simulink model "pulse1"  (R2014b)
settings: Solver=ode45  StartTime=0.0  StopTime=0.5  MaxStep=.00001  RelTol=1e-3
libraries: simulink_extras x6, arduinolib x6, simulink x4, powerlib x1
settings Model: Creator=Muruganandham  LastModifiedBy=SELVA
settings DataIOCC: SignalLoggingSaveFormat=ModelDataLogs
settings OptimizationCC: ExpressionDepthLimit=2147483647
settings DebuggingCC: UnderspecifiedInitializationDetection=Classic  MergeDetectMultiDrivingBlocksExec=none  FcnCallInpInsideContextMsg=UseLocalSettings  StateNameClashWarn=warning
settings GRTTargetCC: CombineOutputUpdateFcns=off  GRTInterface=on

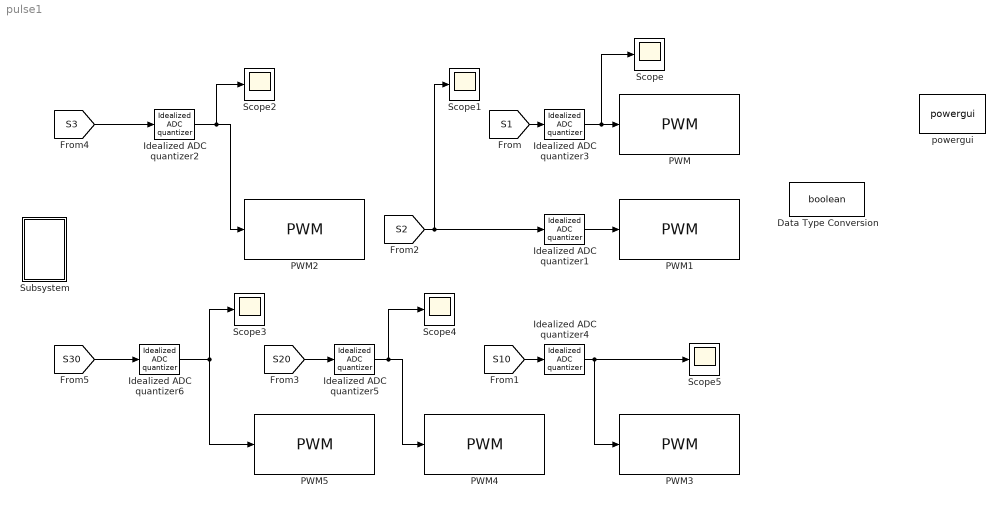
== system pulse1 ==
  Data Type Conversion : DataTypeConversion  OutDataTypeStr=boolean
  Idealized ADC quantizer{1..6} (6 alike) : simulink_extras/Additional Discrete/Idealized ADC quantizer  NumberOfConverterBits=8  Vmin=0  Vmax=5  OutputDataType=int16  OutputNegativeValues=off
  PWM : arduinolib/PWM  pinNumber=2  blockPlatform=arduino
  PWM1 : arduinolib/PWM  pinNumber=3  blockPlatform=arduino
  PWM2 : arduinolib/PWM  pinNumber=4  blockPlatform=arduino
  PWM3 : arduinolib/PWM  pinNumber=5  blockPlatform=arduino
  PWM4 : arduinolib/PWM  pinNumber=6  blockPlatform=arduino
  PWM5 : arduinolib/PWM  pinNumber=6  blockPlatform=arduino
  Scope{,1..5} (6 alike) : Scope
      Scope2 settings: SaveName=ScopeData2
      Scope3 settings: SaveName=ScopeData3
      Scope4 settings: SaveName=ScopeData4
      Scope5 settings: SaveName=ScopeData5
  Subsystem : Subsystem  mask{fc=1000, m=1}
      mask prompts: fc "Switching frequency"; m "modulation index"
  powergui : powerlib/powergui  Priority=1  SimulationMode=Continuous  SolverType=Tustin  SampleTime=50e-6  frequency=60  SPID=off  DisableSnubberDevices=off  DisableRonSwitches=off  DisableVfSwitches=off  SwTol=0  DisplayEquations=off  Interpol=off  methode=off  Ts=0  frequencyindice=0  Pbase=100e6  ErrMax=1e-4  Iterations=50  UnitsV=kV  UnitsW=MW  FunctionMessages=off  echomessages=off  HookPort=off  EnableUseOfTLC=off  x0status=blocks  RestoreLinks=warning  ResistiveCurrentMeasurement=off  Frange=[0:2:500]  Ylog=off  Xlog=on  ShowGrid=off  save=off  variable=ZData  structure=bh  ZoomFFT=off  StartTime=0.0  cycles=50  DisplayStyle=1  fundamental=50  FreqAxis=off  MaxFrequency=1000  frequencyindicesteady=1  RmsSteady=1  display=off
  wires:
  [S1] -> Idealized ADC quantizer3/1
  [S2] -> Scope1/1, Idealized ADC quantizer1/1
  [S3] -> Idealized ADC quantizer2/1
  [S10] -> Idealized ADC quantizer4/1
  [S20] -> Idealized ADC quantizer5/1
  [S30] -> Idealized ADC quantizer6/1
  Idealized ADC quantizer2/1 -> Scope2/1, PWM2/1
  Idealized ADC quantizer1/1 -> PWM1/1
  Idealized ADC quantizer3/1 -> Scope/1, PWM/1
  Idealized ADC quantizer4/1 -> Scope5/1, PWM3/1
  Idealized ADC quantizer5/1 -> Scope4/1, PWM4/1
  Idealized ADC quantizer6/1 -> Scope3/1, PWM5/1

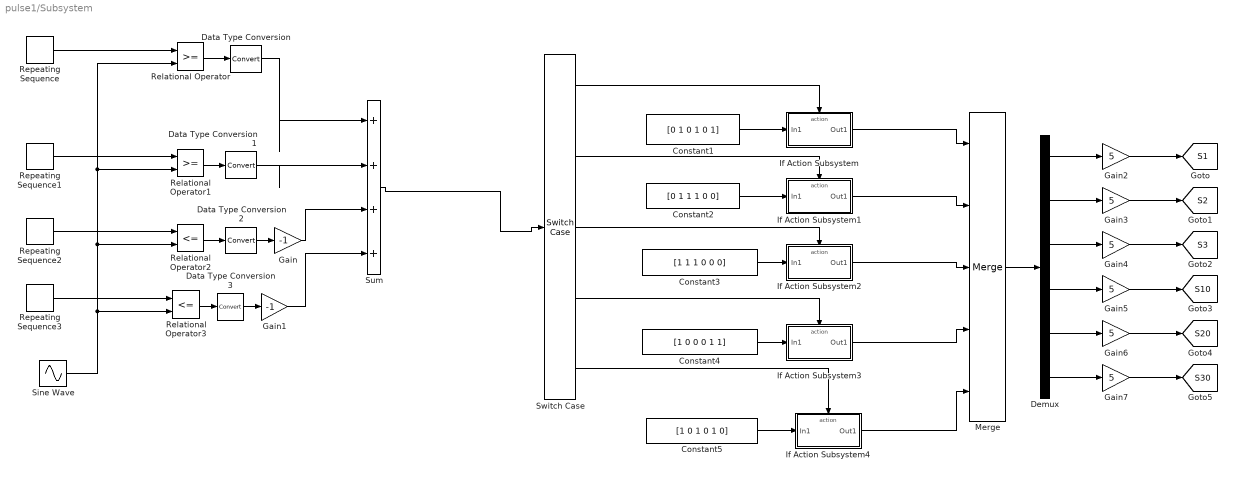
== system pulse1/Subsystem ==
  Constant1 : Constant  Value=[0 1 0 1 0 1]
  Constant2 : Constant  Value=[0 1 1 1 0 0]
  Constant3 : Constant  Value=[1 1 1 0 0 0]
  Constant4 : Constant  Value=[1 0 0 0 1 1]
  Constant5 : Constant  Value=[1 0 1 0 1 0]
  Data Type Conversion{,1..3} (4 alike) : DataTypeConversion
  Demux : Demux  Outputs=6
  Gain : Gain  Gain=-1
  Gain1 : Gain  Gain=-1
  Gain{2..7} (6 alike) : Gain  Gain=5
  If Action Subsystem : Subsystem  TreatAsAtomicUnit=on
  If Action Subsystem1 : Subsystem  TreatAsAtomicUnit=on
  If Action Subsystem2 : Subsystem  TreatAsAtomicUnit=on
  If Action Subsystem3 : Subsystem  TreatAsAtomicUnit=on
  If Action Subsystem4 : Subsystem  TreatAsAtomicUnit=on
  Merge : Merge  Inputs=5
  Relational Operator : RelationalOperator  OutDataTypeStr=boolean
  Relational Operator1 : RelationalOperator  OutDataTypeStr=boolean
  Relational Operator2 : RelationalOperator  Operator=<=  OutDataTypeStr=boolean
  Relational Operator3 : RelationalOperator  Operator=<=  OutDataTypeStr=boolean
  Repeating Sequence : simulink/Sources/Repeating Sequence  rep_seq_t="[0 (1/fc)/2  (1/fc)]"  rep_seq_y=[1 2 1]
  Repeating Sequence1 : simulink/Sources/Repeating Sequence  rep_seq_t="[0 (1/fc)/2  (1/fc)]"  rep_seq_y=[1 0 1]
  Repeating Sequence2 : simulink/Sources/Repeating Sequence  rep_seq_t="[0 (1/fc)/2  (1/fc)]"  rep_seq_y=[-1 0 -1]
  Repeating Sequence3 : simulink/Sources/Repeating Sequence  rep_seq_t="[0 (1/fc)/2  (1/fc)]"  rep_seq_y=[-1 -2 -1]
  Sine Wave : Sin  Amplitude=2*m  Frequency=2*pi*50  SampleTime=0
  Sum : Sum  Inputs=|++++
  Switch Case : SwitchCase  CaseConditions={-2 -1 0 1 2}  ShowDefaultCase=off
  tag scope: S10=global, S1=global, S20=global, S2=global, S30=global, S3=global
  wires:
  Switch Case/5 -> If Action Subsystem4/Action
  Switch Case/4 -> If Action Subsystem3/Action
  Switch Case/3 -> If Action Subsystem2/Action
  Switch Case/2 -> If Action Subsystem1/Action
  Switch Case/1 -> If Action Subsystem/Action
  Constant1/1 -> If Action Subsystem/1(In1)
  Constant2/1 -> If Action Subsystem1/1(In1)
  Constant3/1 -> If Action Subsystem2/1(In1)
  Constant4/1 -> If Action Subsystem3/1(In1)
  Constant5/1 -> If Action Subsystem4/1(In1)
  If Action Subsystem/1(Out1) -> Merge/1
  If Action Subsystem1/1(Out1) -> Merge/2
  If Action Subsystem2/1(Out1) -> Merge/3
  If Action Subsystem3/1(Out1) -> Merge/4
  If Action Subsystem4/1(Out1) -> Merge/5
  Merge/1 -> Demux/1
  Demux/2 -> Gain3/1
  Demux/3 -> Gain4/1
  Demux/4 -> Gain5/1
  Demux/5 -> Gain6/1
  Demux/6 -> Gain7/1
  Relational Operator/1 -> Data Type Conversion/1
  Relational Operator1/1 -> Data Type Conversion1/1
  Gain/1 -> Sum/3
  Gain1/1 -> Sum/4
  Sum/1 -> Switch Case/1
  Repeating Sequence/1 -> Relational Operator/1
  Repeating Sequence1/1 -> Relational Operator1/1
  Repeating Sequence2/1 -> Relational Operator2/1
  Repeating Sequence3/1 -> Relational Operator3/1
  Sine Wave/1 -> Relational Operator1/2, Relational Operator/2, Relational Operator2/2, Relational Operator3/2
  Relational Operator2/1 -> Data Type Conversion2/1
  Relational Operator3/1 -> Data Type Conversion3/1
  Data Type Conversion/1 -> Sum/1
  Data Type Conversion1/1 -> Sum/2
  Data Type Conversion2/1 -> Gain/1
  Data Type Conversion3/1 -> Gain1/1
  Demux/1 -> Gain2/1
  Gain2/1 -> [S1]
  Gain3/1 -> [S2]
  Gain4/1 -> [S3]
  Gain5/1 -> [S10]
  Gain6/1 -> [S20]
  Gain7/1 -> [S30]

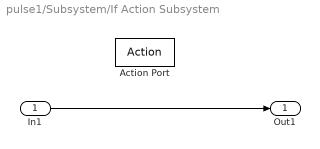
== system pulse1/Subsystem/If Action Subsystem ==
  In1 : Inport
  Action Port : ActionPort  ActionType=case
  Out1 : Outport
  wires:
  In1/1 -> Out1/1

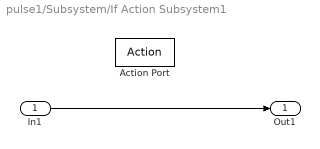
== system pulse1/Subsystem/If Action Subsystem1 ==
  In1 : Inport
  Action Port : ActionPort  ActionType=case
  Out1 : Outport
  wires:
  In1/1 -> Out1/1

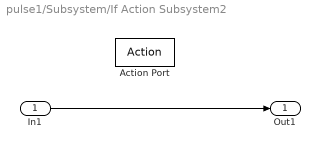
== system pulse1/Subsystem/If Action Subsystem2 ==
  In1 : Inport
  Action Port : ActionPort  ActionType=case
  Out1 : Outport
  wires:
  In1/1 -> Out1/1

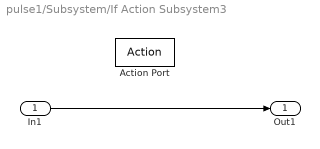
== system pulse1/Subsystem/If Action Subsystem3 ==
  In1 : Inport
  Action Port : ActionPort  ActionType=case
  Out1 : Outport
  wires:
  In1/1 -> Out1/1

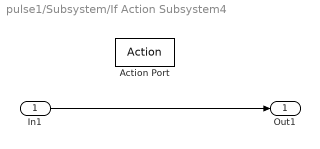
== system pulse1/Subsystem/If Action Subsystem4 ==
  In1 : Inport
  Action Port : ActionPort  ActionType=case
  Out1 : Outport
  wires:
  In1/1 -> Out1/1
